simulink model "SimElectronics_DC_Motor_SPE_START"  (R2016b)
settings: Solver=ode15s  StartTime=0.0  StopTime=4  RelTol=1e-3  EnableMultiTasking=on
PreLoadFcn:
  | load SimElectronics_DC_Motor_SPE_Data;
  | load SimElectronics_DC_Motor_SPE_Param_Start;
undefined symbols (not defined in the file or in its folder): DC_Motor_J
libraries: fl_lib x15, nesl_utility x6, elec_lib x1
Description:
  | Copyright 2014 The MathWorks, Inc.
settings Model: Creator=smiller  LastModifiedBy=gd7198
settings DataIOCC: ExternalInput=[SS_DC_Motor_SPE_Input_time SS_DC_Motor_SPE_Input_Signal]  LimitDataPoints=on  LoadExternalInput=on  SaveFormat=Array
settings OptimizationCC: ExpressionDepthLimit=2147483647  InitFltsAndDblsToZero=on  LifeSpan=inf
settings DebuggingCC: SaveWithParameterizedLinksMsg=none  UnderspecifiedInitializationDetection=Classic  MergeDetectMultiDrivingBlocksExec=none  FcnCallInpInsideContextMsg=warning  StateNameClashWarn=warning  SFUnexpectedBacktrackingDiag=warning  SFNoUnconditionalDefaultTransitionDiag=warning  SFExecutionAtInitializationDiag=none
settings HardwareCC: ProdBitPerPointer=32  ProdBitPerSizeT=32  ProdBitPerPtrDiffT=32  ProdLargestAtomicFloat=None  ProdIntDivRoundTo=Undefined  ProdEndianess=Unspecified  ProdWordSize=32  ProdHWDeviceType=32-bit Generic
settings ModelReferenceCC: PropagateSignalLabelsOutOfModel=off
settings GRTTargetCC: TargetFcnLib=ansi_tfl_tmw.mat  TargetLangStandard=C89/C90 (ANSI)  GeneratePreprocessorConditionals=Disable all  CombineOutputUpdateFcns=off  GRTInterface=on
settings ConfigComp: CovMetricSettings=dw  CovHtmlReporting=on  CovSaveCumulativeToWorkspaceVar=on  CovSaveSingleToWorkspaceVar=on  CovExternalEMLEnable=off  CovSFcnEnable=off

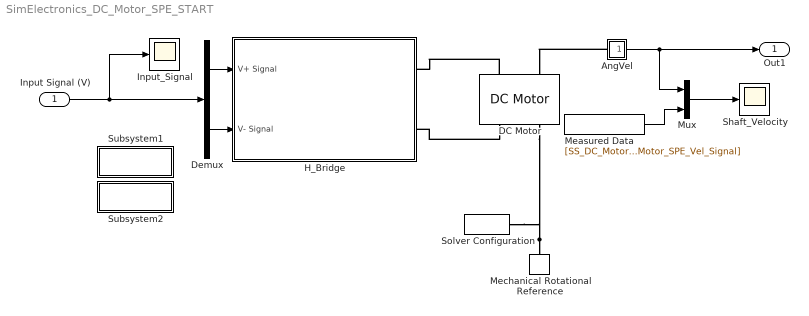
== system SimElectronics_DC_Motor_SPE_START ==
  Input Signal (V) : Inport  PortDimensions=2
  AngVel : Subsystem  Description=Simscape Probe  InitFcn=|
      | unit=get_param([gcb '/PS-S'],'Unit');                                              
      | set_param(gcb, 'AttributesFormatString', strcat('[', unit,']'));
      mask help: Simscape Probe
      settings: AttributesFormatString=[rad/s]
      settings: CopyFcn=|
      | set_param(gcb,'LinkStatus','inactive');
      | set_param(gcb,'LinkStatus','none');
      | set_param([gcb '/Goto'],'GotoTag', [get(gcbh,'name')]);
      | set_param([gcb '/From'],'GotoTag', [get(gcbh,'name')]);
      | h = get_param([gcb, '/PS-S'], 'PortHandles');
      | set(h.Outport(1), 'SignalNameFromLabel', [get(gcbh,'name')])
      | clear h;
      settings: NameChangeFcn=|
      | set_param([gcb '/Goto'],'GotoTag', [get(gcbh,'name')]);
      | set_param([gcb '/From'],'GotoTag', [get(gcbh,'name')]);
      | h = get_param([gcb, '/PS-S'], 'PortHandles');
      | set(h.Outport(1), 'SignalNameFromLabel', [get(gcbh,'name')])
      | clear h;
      settings: OpenFcn=|
      | if exist('logsout', 'var')
      |   vname = get(gcbh,'name');
      |   fHandle = findall(0,'Tag',vname);
      |   if isempty(fHandle)
      |   figure('Tag',vname);
      |   end;
      |   figure(findobj('Tag',vname));
      |   plot(logsout.getElement([gcb, '/PS-S'], '-blockpath').Values)
      |   title(get(gcbh,'name'));
      |   ylabel(['Anguiar Velocity (' get_param([gcb '/PS-S'],'Unit') ')'] );
      | end
      mask Display: port_label('LConn', 1,'\omega','texmode', 'on');
  DC Motor : elec_lib/Actuators & Drivers/Rotational Actuators/DC Motor  parameterization=1  Ra=DC_Motor_R Ohm  La=DC_Motor_L H  emf_or_torque=1  Kv=DC_Motor_K V/(rad/s)  Ki=6.876e-4 N*m/A  T_stall=2.4e-4 N*m  w_max=1.91e+4 rpm  w_rated=1.5e+4 rpm  P_rated=0.08 W  V_rated=1.5 V  J=DC_Motor_J kg*m^2  lam_param=1  lam=DC_Motor_B N*m/(rad/s)  i_noload=0 A  V_i_noload=1.5 V  speed0=0 rpm  alpha=0.00393 1/K  Tmeas=25 C  thermal_mass=100 J/K  initial_temperature=25 C
  Demux : Demux  Outputs=2
  H_Bridge : Subsystem
      mask Display:
      | image(imread('H_Bridge.jpg'));
      | port_label('Input',1,'V+ Signal');
      | port_label('Input',2,'V- Signal');
      | port_label('rconn',1,'V+');
      | port_label('rconn',2,'V-');
  Input_Signal : Scope
  Measured Data : FromWorkspace  VariableName=[SS_DC_Motor_SPE_Vel_time SS_DC_Motor_SPE_Vel_Signal]  SampleTime=0
  Mechanical Rotational Reference : fl_lib/Mechanical/Rotational Elements/Mechanical Rotational Reference
  Mux : Mux  Inputs=2
  Shaft_Velocity : Scope
  Solver Configuration : nesl_utility/Solver Configuration  PhysicalDomain=network_engine_domain  SubClassName=solver  LeftPortType=input  RightPortType=generic  Accelerate=off  Tones=[]  Harmonics=[]  SimulateNoise=off  Profile=off  UseLocalSampling=off  EnableSwitchedLinearOptims=on  FrequencyDomain=off  UseCCode=off  RelTol=0.001  AbsTol=1e-06  MinStep=1e-09  ToWorkspace=off  RevertToSquareIcSolve=off  NumHomotopyIterations=100  PhasorMode=off  PhasorModeNumHarmonics=1  OverrideAbsTol=off  DoDC=off  ResidualTolerance=1e-9  UseLocalSolver=off  LocalSolverChoice=NE_BACKWARD_EULER_ADVANCER  LocalSolverSampleTime=.001  DoFixedCost=off  MaxNonlinIter=12  MaxModeIter=1  LinearAlgebra=Sparse  DelaysMemoryBudget=1024  AutomaticFiltering=on  FilteringTimeConstant=0.001
  Subsystem1 : Subsystem
      settings: OpenFcn=load SimElectronics_DC_Motor_SPE_Param_Start;
      mask Display: disp('Orig. Values')
  Subsystem2 : Subsystem
      settings: OpenFcn=load SimElectronics_DC_Motor_SPE_Param_Final;
      mask Display: disp('Final Values')
  Out1 : Outport
  wires:
  Input Signal (V)/1 -> Demux/1, Input_Signal/1
  Demux/1 -> H_Bridge/1(V+ Signal)
  Demux/2 -> H_Bridge/2(V- Signal)
  Mux/1 -> Shaft_Velocity/1
  Measured Data/1 -> Mux/2
  AngVel/1(Out) -> Out1/1, Mux/1
  connections:
  Mechanical Rotational Reference/LConn1 -- DC Motor/RConn2 -- Solver Configuration/RConn1
  DC Motor/LConn1 -- H_Bridge/RConn1
  DC Motor/RConn1 -- H_Bridge/RConn2
  AngVel/LConn1 -- DC Motor/LConn2

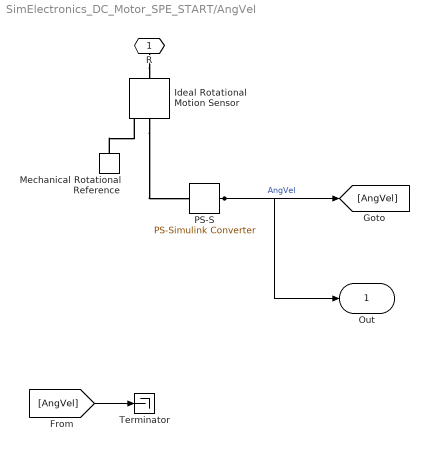
== system SimElectronics_DC_Motor_SPE_START/AngVel ==
  Ideal Rotational Motion Sensor : fl_lib/Mechanical/Mechanical Sensors/Ideal Rotational Motion Sensor  offset=0 rad
  Mechanical Rotational Reference : fl_lib/Mechanical/Rotational Elements/Mechanical Rotational Reference
  PS-S : nesl_utility/PS-Simulink Converter  PhysicalDomain=network_engine_domain  SubClassName=ps_output  LeftPortType=input  RightPortType=output  PseudoPeriodic=off  Frequencies=[]  Unit=rad/s  AffineConversion=off
  Terminator : Terminator
  R : PMIOPort  Port=1  Side=Left
  Out : Outport
  wires:
  [AngVel] -> Terminator/1
  PS-S/1 -> [AngVel], Out/1  "AngVel"
  connections:
  R/RConn1 -- Ideal Rotational Motion Sensor/LConn1
  Mechanical Rotational Reference/LConn1 -- Ideal Rotational Motion Sensor/RConn1
  Ideal Rotational Motion Sensor/RConn2 -- PS-S/LConn1

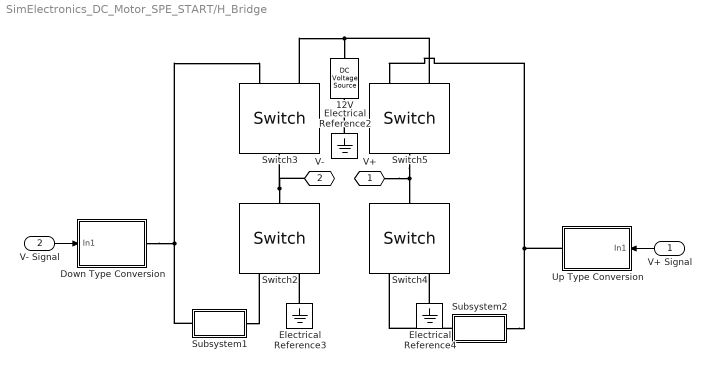
== system SimElectronics_DC_Motor_SPE_START/H_Bridge ==
  V+ Signal : Inport
  V- Signal : Inport  Port=2
  12V : fl_lib/Electrical/Electrical Sources/DC Voltage Source  v0=12 V
  Down Type Conversion : Subsystem
  Electrical Reference2 : fl_lib/Electrical/Electrical Elements/Electrical Reference
  Electrical Reference3 : fl_lib/Electrical/Electrical Elements/Electrical Reference
  Electrical Reference4 : fl_lib/Electrical/Electrical Elements/Electrical Reference
  Subsystem1 : Subsystem
      mask Display: disp('NOT');
  Subsystem2 : Subsystem
      mask Display: disp('NOT');
  Switch{2..5} (4 alike) : fl_lib/Electrical/Electrical Elements/Switch  R_closed=0.01 Ohm  G_open=1e-8 1/Ohm  Threshold=0  i_specify=off  i_priority=High  i=0 A  v_specify=off  v_priority=High  v=0 V
  Up Type Conversion : Subsystem
  V+ : PMIOPort  Port=1  Side=Right
  V- : PMIOPort  Port=2  Side=Right
  wires:
  V+ Signal/1 -> Up Type Conversion/1(In1)
  V- Signal/1 -> Down Type Conversion/1(In1)
  connections:
  Up Type Conversion/RConn1 -- Switch5/RConn1 -- Subsystem2/LConn1
  Subsystem2/RConn1 -- Switch4/RConn1
  Electrical Reference4/LConn1 -- Switch4/RConn2
  Subsystem1/RConn1 -- Switch2/RConn1
  Electrical Reference3/LConn1 -- Switch2/RConn2
  Electrical Reference2/LConn1 -- 12V/RConn1
  Switch2/LConn1 -- Switch3/LConn1 -- V-/RConn1
  Down Type Conversion/RConn1 -- Switch3/RConn1 -- Subsystem1/LConn1
  Switch5/RConn2 -- 12V/LConn1 -- Switch3/RConn2
  Switch5/LConn1 -- Switch4/LConn1 -- V+/RConn1

== system SimElectronics_DC_Motor_SPE_START/Subsystem1 ==

== system SimElectronics_DC_Motor_SPE_START/Subsystem2 ==

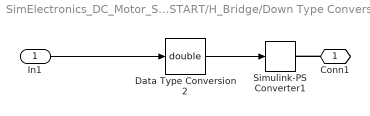
== system SimElectronics_DC_Motor_SPE_START/H_Bridge/Down Type Conversion ==
  In1 : Inport
  Data Type Conversion2 : DataTypeConversion  OutDataTypeStr=double
  Simulink-PS Converter1 : nesl_utility/Simulink-PS Converter  PhysicalDomain=network_engine_domain  SubClassName=ps_input  LeftPortType=input  RightPortType=output  PseudoPeriodic=off  Frequencies=[]  NoiseDistribution=none  NoiseParameters=[]  Unit=1  AffineConversion=off  InputFiltering=off  SimscapeFilterOrder=1  InputFilterTimeConstant=.001  UdotUserProvided=0
  Conn1 : PMIOPort  Port=1  Side=Right
  wires:
  Data Type Conversion2/1 -> Simulink-PS Converter1/1
  In1/1 -> Data Type Conversion2/1
  connections:
  Conn1/RConn1 -- Simulink-PS Converter1/RConn1

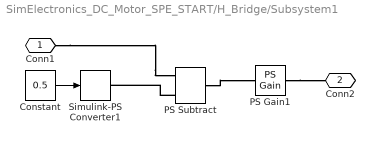
== system SimElectronics_DC_Motor_SPE_START/H_Bridge/Subsystem1 ==
  Constant : Constant  Value=0.5
  PS Gain1 : fl_lib/Physical Signals/Functions/PS Gain  gain=-1
  PS Subtract : fl_lib/Physical Signals/Functions/PS Subtract
  Simulink-PS Converter1 : nesl_utility/Simulink-PS Converter  PhysicalDomain=network_engine_domain  SubClassName=ps_input  LeftPortType=input  RightPortType=output  PseudoPeriodic=off  Frequencies=[]  NoiseDistribution=none  NoiseParameters=[]  Unit=1  AffineConversion=off  InputFiltering=off  SimscapeFilterOrder=1  InputFilterTimeConstant=.001  UdotUserProvided=0
  Conn1 : PMIOPort  Port=1  Side=Left
  Conn2 : PMIOPort  Port=2  Side=Right
  wires:
  Constant/1 -> Simulink-PS Converter1/1
  connections:
  PS Subtract/LConn2 -- Simulink-PS Converter1/RConn1
  Conn1/RConn1 -- PS Subtract/LConn1
  PS Subtract/RConn1 -- PS Gain1/LConn1
  PS Gain1/RConn1 -- Conn2/RConn1

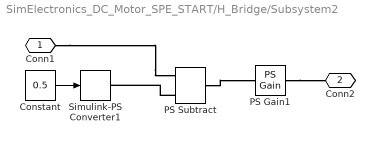
== system SimElectronics_DC_Motor_SPE_START/H_Bridge/Subsystem2 ==
  Constant : Constant  Value=0.5
  PS Gain1 : fl_lib/Physical Signals/Functions/PS Gain  gain=-1
  PS Subtract : fl_lib/Physical Signals/Functions/PS Subtract
  Simulink-PS Converter1 : nesl_utility/Simulink-PS Converter  PhysicalDomain=network_engine_domain  SubClassName=ps_input  LeftPortType=input  RightPortType=output  PseudoPeriodic=off  Frequencies=[]  NoiseDistribution=none  NoiseParameters=[]  Unit=1  AffineConversion=off  InputFiltering=off  SimscapeFilterOrder=1  InputFilterTimeConstant=.001  UdotUserProvided=0
  Conn1 : PMIOPort  Port=1  Side=Left
  Conn2 : PMIOPort  Port=2  Side=Right
  wires:
  Constant/1 -> Simulink-PS Converter1/1
  connections:
  PS Gain1/RConn1 -- Conn2/RConn1
  PS Subtract/RConn1 -- PS Gain1/LConn1
  Conn1/RConn1 -- PS Subtract/LConn1
  PS Subtract/LConn2 -- Simulink-PS Converter1/RConn1

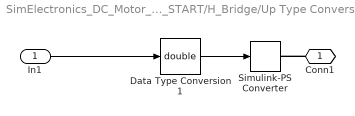
== system SimElectronics_DC_Motor_SPE_START/H_Bridge/Up Type Conversion ==
  In1 : Inport
  Data Type Conversion1 : DataTypeConversion  OutDataTypeStr=double
  Simulink-PS Converter : nesl_utility/Simulink-PS Converter  PhysicalDomain=network_engine_domain  SubClassName=ps_input  LeftPortType=input  RightPortType=output  PseudoPeriodic=off  Frequencies=[]  NoiseDistribution=none  NoiseParameters=[]  Unit=1  AffineConversion=off  InputFiltering=off  SimscapeFilterOrder=1  InputFilterTimeConstant=.001  UdotUserProvided=0
  Conn1 : PMIOPort  Port=1  Side=Right
  wires:
  Data Type Conversion1/1 -> Simulink-PS Converter/1
  In1/1 -> Data Type Conversion1/1
  connections:
  Conn1/RConn1 -- Simulink-PS Converter/RConn1
